simulink model "SF103A_MotRefMdl"  (R2013b)
settings: Solver=FixedStepDiscrete  StartTime=0.0  StopTime=2  FixedStep=.002  RelTol=1e-3
values from neighbouring files (symbols this model uses):
  ARCHGLBPRM_2MILLISEC_SEC_F32 = DataDict.Constant    [SF103A_MotRefMdl_DataDict.m]
  ARCHGLBPRM_2OVERSQRT3_ULS_F32 = DataDict.Constant    [SF103A_MotRefMdl_DataDict.m]
  ARCHGLBPRM_2PI_ULS_F32 = DataDict.Constant    [SF103A_MotRefMdl_DataDict.m]
  ARCHGLBPRM_4OVERSQRT3_ULS_F32 = DataDict.Constant    [SF103A_MotRefMdl_DataDict.m]
  ARCHGLBPRM_5PIOVER4_ULS_F32 = DataDict.Constant    [SF103A_MotRefMdl_DataDict.m]
  ARCHGLBPRM_FLOATZEROTHD_ULS_F32 = DataDict.Constant    [SF103A_MotRefMdl_DataDict.m]
  ARCHGLBPRM_HALFSQRT3_ULS_F32 = DataDict.Constant    [SF103A_MotRefMdl_DataDict.m]
  ARCHGLBPRM_PI_ULS_F32 = DataDict.Constant    [SF103A_MotRefMdl_DataDict.m]
  MotRefMdlCurrDaxBoostGain = DataDict.Calibration    [SF103A_MotRefMdl_DataDict.m]
  MotRefMdlCurrDaxQaxRefDelta = DataDict.Calibration    [SF103A_MotRefMdl_DataDict.m]
  MotRefMdlCurrItrnTolr = DataDict.Calibration    [SF103A_MotRefMdl_DataDict.m]
  MotRefMdlFbCtrlDi = DataDict.Calibration    [SF103A_MotRefMdl_DataDict.m]
  MotRefMdlIvtrDeadTiBrdgVltgSca = DataDict.Calibration    [SF103A_MotRefMdl_DataDict.m]
  MotRefMdlMinCurrItrnLim = DataDict.Calibration    [SF103A_MotRefMdl_DataDict.m]
  MotRefMdlMotCurrDaxMaxSca = DataDict.Calibration    [SF103A_MotRefMdl_DataDict.m]
  MotRefMdlMotVltgDerivtvTiCon = DataDict.Calibration    [SF103A_MotRefMdl_DataDict.m]
  MotRefMdlRefLocnItrnLim = DataDict.Calibration    [SF103A_MotRefMdl_DataDict.m]
  MotRefMdlTqItrnLim = DataDict.Calibration    [SF103A_MotRefMdl_DataDict.m]
  MotRefMdlTqItrnTolr = DataDict.Calibration    [SF103A_MotRefMdl_DataDict.m]
  MotRefMdlVltgModDynCmpEna = DataDict.Calibration    [SF103A_MotRefMdl_DataDict.m]
  MotRefMdlVltgOverRThdSca = DataDict.Calibration    [SF103A_MotRefMdl_DataDict.m]
  SysGlbPrmMotPoleCnt = DataDict.ImprtdCal    [SF103A_MotRefMdl_DataDict.m]
undefined symbols (not defined in the file or in its folder): MotQuad1
libraries: NxtrLim x19, simulink x4, LnrIntrpn x3, Fil x2, NxtrAbslt x2, FixdToFloat x2, FloatToFixd x2, NxtrMath x1
(part 4 of 7)

== system SF103A_MotRefMdl/MotRefMdl/MotRefMdlPer1/DAxisCurrentBoost/If Action Subsystem ==
  note: "VoltageMargin"
  note: "Vmag_min/R"
  CurrDaxMin : Inport  RequirementInfo={} %GIDa_a9cc6c0e_d971_41b8_a873_ef9f53fa8bc6
  CurrQaxMin : Inport  RequirementInfo={} %GIDa_a98a38c5_8ae3_4bcc_9086_28c16690a326  Port=2
  InterCalcns : Inport  RequirementInfo={} %GIDa_5e92023f_1a23_4fc8_ae94_2c4b8c4c5d26  Port=3
  MotTqCmdLimd : Inport  Port=4
  CurrDaxAtPeakTq : Inport  Port=5
  Action Port : ActionPort  ActionType=then
  Add : Sum  RequirementInfo={'linktype_rmi_doors' '0000bb42 (/E-STEER Core/SubSystem Specifications/Application Functions/SF99/SF103A Motor Reference Model)' '#SF103A_142' 'true' 'REQ:SF103A_142' '' } %GIDa_a7207258_8a7c_4a3a_8c14_f88ec2ccdf28
  Boost_Merge : Merge  RequirementInfo={'linktype_rmi_doors' '0000bb42 (/E-STEER Core/SubSystem Specifications/Application Functions/SF99/SF103A Motor Reference Model)' '#SF103A_145' 'true' 'REQ:SF103A_145' '' } %GIDa_8158cc00_aa92_4509_984e_a32d4237c8b1
  Bus Selector : BusSelector  RequirementInfo={} %GIDa_f3165034_7368_454c_b0f7_31404390f148  OutputSignals=VltgOverR_Ampr
  Constant : Constant  RequirementInfo={'linktype_rmi_doors' '0000bb42 (/E-STEER Core/SubSystem Specifications/Application Functions/SF99/SF103A Motor Reference Model)' '#SF103A_143' 'true' 'REQ:SF103A_143' '' } %GIDa_b9afd42a_ca58_4d6b_8dd6_d9cdb6968168  Value=MotRefMdlVltgOverRThdSca
  Constant1 : Constant  RequirementInfo={'linktype_rmi_doors' '0000bb42 (/E-STEER Core/SubSystem Specifications/Application Functions/SF99/SF103A Motor Reference Model)' '#SF103A_145' 'true' 'REQ:SF103A_145' '' } %GIDa_acfabe03_75a7_44a2_9eb9_3f49c5171f7f  Value=0  OutDataTypeStr=single
  CopyRight2 : Subsystem  Description=|  mask(Copyright Information){none=on}
      | Copyright info block.                                               
      |                                                                     
      | Place copyright information at the top of every subsystem in design.
      mask prompts: none "No parameters"
      mask help: Place copyright information at the top of every subsystem in design.
      mask Display:
      | NxtrConf = 'Nexteer Confidential';
      | 
      | sys = bdroot; %handle for the current model ("system")
      | first = get_param(sys,'Created');
      | first = first(end-3:end);  %year is last four digits
      | 
      | last = get_param(sys,'LastModifiedDate');
      | if isempty(last)
      |     last = datestr(now,'yyyy');
      | else
      |     last = last(end-3:end);
      | end
      | 
      | if strcmp(first,last)
      |     fprintf('%s -- Copyright %s Nexteer',NxtrConf,first)
      | else
      |     fprintf('%s -- %s%s- %s Nexteer',NxtrConf,char(169),first,last)
      | end
  "CurrToVoltTest " : Subsystem
  Dax_Merge : Merge  RequirementInfo={'linktype_rmi_doors' '0000bb42 (/E-STEER Core/SubSystem Specifications/Application Functions/SF99/SF103A Motor Reference Model)' '#SF103A_145' 'true' 'REQ:SF103A_145' '' } %GIDa_3f0604bd_3f78_4abe_886a_80594115c85c
  If : If  RequirementInfo={'linktype_rmi_doors' '0000bb42 (/E-STEER Core/SubSystem Specifications/Application Functions/SF99/SF103A Motor Reference Model)' '#SF103A_145' 'true' 'REQ:SF103A_145' '' ; 'linktype_rmi_doors' '0000bb42 (/E-STEER Core/SubSystem Specifications/Application Functions/SF99/SF103A Motor Reference Model)' '#SF103A_149' 'true' 'REQ:SF103A_149' '' } %GIDa_18434ab9_b410_43c2_a56e_97fbbcb99bff  IfExpression=u1 >= 0
  If Action Subsystem : Subsystem  RequirementInfo={'linktype_rmi_doors' '0000bb42 (/E-STEER Core/SubSystem Specifications/Application Functions/SF99/SF103A Motor Reference Model)' '#SF103A_149' 'true' 'REQ:SF103A_149' '' } %GIDa_5e584c9f_7420_4cd1_86a2_c32478ec1f58  TreatAsAtomicUnit=on
  Math Function : Math  RequirementInfo={'linktype_rmi_doors' '0000bb42 (/E-STEER Core/SubSystem Specifications/Application Functions/SF99/SF103A Motor Reference Model)' '#SF103A_142' 'true' 'REQ:SF103A_142' '' } %GIDa_7944bbab_6b21_43ee_b623_3ef25e5888e6  Operator=square  SaturateOnIntegerOverflow=on
  Math Function1 : Math  RequirementInfo={'linktype_rmi_doors' '0000bb42 (/E-STEER Core/SubSystem Specifications/Application Functions/SF99/SF103A Motor Reference Model)' '#SF103A_142' 'true' 'REQ:SF103A_142' '' } %GIDa_493eb05e_2677_4cd4_acc7_ad4c5e79bd89  Operator=square  SaturateOnIntegerOverflow=on
  Product : Product  RequirementInfo={'linktype_rmi_doors' '0000bb42 (/E-STEER Core/SubSystem Specifications/Application Functions/SF99/SF103A Motor Reference Model)' '#SF103A_143' 'true' 'REQ:SF103A_143' '' } %GIDa_05a785fc_6d2b_42f5_8278_a505a2fee388  RndMeth=Zero
  Qax_Merge : Merge  RequirementInfo={'linktype_rmi_doors' '0000bb42 (/E-STEER Core/SubSystem Specifications/Application Functions/SF99/SF103A Motor Reference Model)' '#SF103A_145' 'true' 'REQ:SF103A_145' '' } %GIDa_c18f4407_faf9_46c8_81f8_a25da43b62c9
  Sqrt_f32 : NxtrMath/Sqrt_f32  SFunctionSpec=single y1 = Sqrt_f32(single u1)  ShowSpec=off
      settings: AttributesFormatString=%<MaskType>
  Subtract : Sum  RequirementInfo={'linktype_rmi_doors' '0000bb42 (/E-STEER Core/SubSystem Specifications/Application Functions/SF99/SF103A Motor Reference Model)' '#SF103A_143' 'true' 'REQ:SF103A_143' '' } %GIDa_ee97ca05_4079_4b26_a98f_acc77e80c0bc  Inputs=+-
  pass_thru : Subsystem  RequirementInfo={'linktype_rmi_doors' '0000bb42 (/E-STEER Core/SubSystem Specifications/Application Functions/SF99/SF103A Motor Reference Model)' '#SF103A_145' 'true' 'REQ:SF103A_145' '' } %GIDa_4f4a4179_c5b2_4767_8ef4_f1533bcda9c5  TreatAsAtomicUnit=on
  CurrDaxBoostd : Outport  RequirementInfo={} %GIDa_c7761a80_f9a5_4df9_8815_ca0dff25a232
  CurrQaxBoostd : Outport  RequirementInfo={} %GIDa_0eb399b5_a76d_490b_968a_f2f0f65fb18a  Port=2
  BoostAmnt : Outport  RequirementInfo={} %GIDa_326380c9_363e_48c7_b65c_8aa2d98ec125  Port=3
  wires:
  Math Function1/1 -> Add/2
  Math Function/1 -> Add/1
  Sqrt_f32/1 -> Subtract/1
  Product/1 -> Subtract/2
  Add/1 -> Sqrt_f32/1  "VRBoostTotal_AmpSq"
  "CurrToVoltTest "/1(VdR_Amp) -> Math Function/1
  Subtract/1 -> If Action Subsystem/1(VRDelta), If/1  "VRDelta_Amp"
  Constant/1 -> Product/2
  "CurrToVoltTest "/2(VqR_Amp) -> Math Function1/1
  Bus Selector/1 -> Product/1  "<VltgOverR_Ampr>"
  [IqMin] -> "CurrToVoltTest "/2(IqRef_Amp)
  InterCalcns/1 -> If Action Subsystem/2(InterCalcns), Bus Selector/1, "CurrToVoltTest "/3(InterCalcns)
  MotTqCmdLimd/1 -> If Action Subsystem/4(MotTqCmdLimd)
  If/1 -> If Action Subsystem/Action
  CurrDaxAtPeakTq/1 -> If Action Subsystem/5(CurrDaxAtPeakTq)
  If/2 -> pass_thru/Action
  [IdMin] -> "CurrToVoltTest "/1(IdRef_Amp)
  CurrDaxMin/1 -> [IdMin]
  [IdMin] -> If Action Subsystem/3(CurrDaxMin)
  Constant1/1 -> pass_thru/1(In1)
  [IdMin] -> pass_thru/2(In2)
  pass_thru/1(Out1) -> Boost_Merge/1
  If Action Subsystem/1(CurrDaxBoostAmnt) -> Boost_Merge/2
  pass_thru/2(Out2) -> Dax_Merge/1
  If Action Subsystem/2(CurrDaxBoostd) -> Dax_Merge/2
  pass_thru/3(Out3) -> Qax_Merge/1
  If Action Subsystem/3(CurrQaxMin) -> Qax_Merge/2
  Dax_Merge/1 -> CurrDaxBoostd/1
  Qax_Merge/1 -> CurrQaxBoostd/1
  Boost_Merge/1 -> BoostAmnt/1
  CurrQaxMin/1 -> [IqMin]
  [IqMin] -> pass_thru/3(In3)

== system SF103A_MotRefMdl/MotRefMdl/MotRefMdlPer1/DAxisCurrentBoost/pass_thru ==
  In1 : Inport
  In2 : Inport  Port=2
  In3 : Inport  Port=3
  Action Port : ActionPort  ActionType=else
  Out1 : Outport
  Out2 : Outport  Port=2
  Out3 : Outport  Port=3
  wires:
  In1/1 -> Out1/1
  In2/1 -> Out2/1
  In3/1 -> Out3/1

== system SF103A_MotRefMdl/MotRefMdl/MotRefMdlPer1/FeedforwardVoltage/CopyRight2 ==

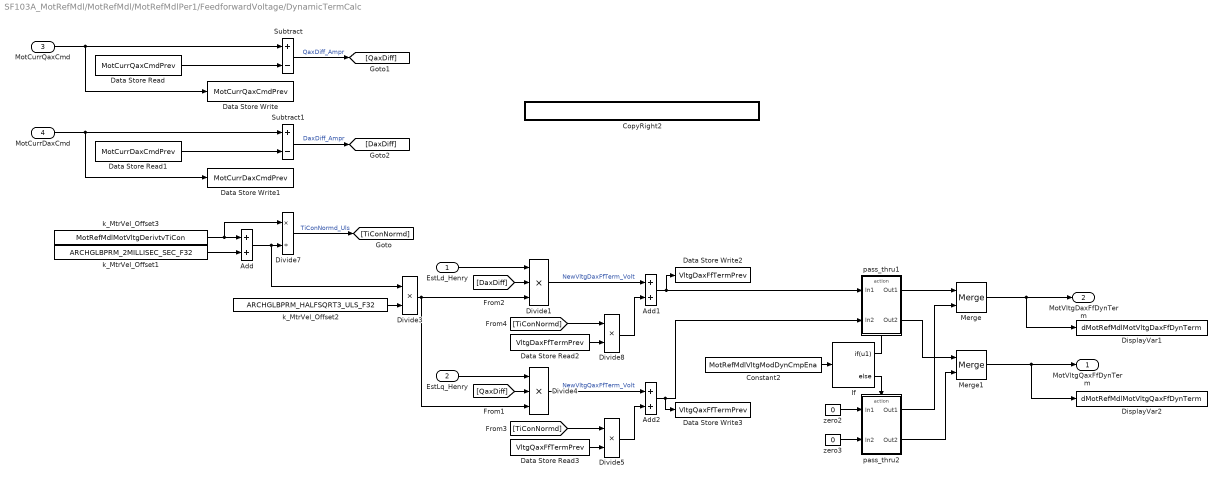
== system SF103A_MotRefMdl/MotRefMdl/MotRefMdlPer1/FeedforwardVoltage/DynamicTermCalc ==
  EstLd_Henry : Inport  RequirementInfo={} %GIDa_669719cb_8e2d_4183_8cde_e2bfb5c3b721
  EstLq_Henry : Inport  RequirementInfo={} %GIDa_1e6f10ed_a02a_410d_b0f0_b2b8d69bc7d9  Port=2
  MotCurrQaxCmd : Inport  RequirementInfo={} %GIDa_48fec4ba_508b_4013_ad2a_d4908a6c34f1  Port=3
  MotCurrDaxCmd : Inport  RequirementInfo={} %GIDa_f1550487_6b07_4eb4_b5b5_ba3d330502de  Port=4
  Add : Sum  RequirementInfo={'linktype_rmi_doors' '0000bb42 (/E-STEER Core/SubSystem Specifications/Application Functions/SF99/SF103A Motor Reference Model)' '#SF103A_160' 'true' 'REQ:SF103A_160' '' ; 'linktype_rmi_doors' '0000bb42 (/E-STEER Core/SubSystem Specifications/Application Functions/SF99/SF103A Motor Reference Model)' '#SF103A_182' 'true' 'REQ:SF103A_182' '' } %GIDa_10232317_d51a_444c_8610_964f10878767
  Add1 : Sum  RequirementInfo={'linktype_rmi_doors' '0000bb42 (/E-STEER Core/SubSystem Specifications/Application Functions/SF99/SF103A Motor Reference Model)' '#SF103A_160' 'true' 'REQ:SF103A_160' '' ; 'linktype_rmi_doors' '0000bb42 (/E-STEER Core/SubSystem Specifications/Application Functions/SF99/SF103A Motor Reference Model)' '#SF103A_182' 'true' 'REQ:SF103A_182' '' } %GIDa_669d8608_a4e4_4a27_aa85_1b2fde54e24b
  Add2 : Sum  RequirementInfo={'linktype_rmi_doors' '0000bb42 (/E-STEER Core/SubSystem Specifications/Application Functions/SF99/SF103A Motor Reference Model)' '#SF103A_160' 'true' 'REQ:SF103A_160' '' ; 'linktype_rmi_doors' '0000bb42 (/E-STEER Core/SubSystem Specifications/Application Functions/SF99/SF103A Motor Reference Model)' '#SF103A_182' 'true' 'REQ:SF103A_182' '' } %GIDa_7f87b368_be3e_4799_a4ca_a1b629f831da
  Constant2 : Constant  RequirementInfo={'linktype_rmi_doors' '0000bb42 (/E-STEER Core/SubSystem Specifications/Application Functions/SF99/SF103A Motor Reference Model)' '#SF103A_181' 'true' 'REQ:SF103A_181' '' } %GIDa_cceb1647_a34e_4756_8fd2_7c70dafabde3  Value=MotRefMdlVltgModDynCmpEna
  CopyRight2 : Subsystem  Description=|  mask(Copyright Information){none=on}
      | Copyright info block.                                               
      |                                                                     
      | Place copyright information at the top of every subsystem in design.
      mask prompts: none "No parameters"
      mask help: Place copyright information at the top of every subsystem in design.
      mask Display:
      | NxtrConf = 'Nexteer Confidential';
      | 
      | sys = bdroot; %handle for the current model ("system")
      | first = get_param(sys,'Created');
      | first = first(end-3:end);  %year is last four digits
      | 
      | last = get_param(sys,'LastModifiedDate');
      | if isempty(last)
      |     last = datestr(now,'yyyy');
      | else
      |     last = last(end-3:end);
      | end
      | 
      | if strcmp(first,last)
      |     fprintf('%s -- Copyright %s Nexteer',NxtrConf,first)
      | else
      |     fprintf('%s -- %s%s- %s Nexteer',NxtrConf,char(169),first,last)
      | end
  Data Store Read : DataStoreRead  RequirementInfo={'linktype_rmi_doors' '0000bb42 (/E-STEER Core/SubSystem Specifications/Application Functions/SF99/SF103A Motor Reference Model)' '#SF103A_160' 'true' 'REQ:SF103A_160' '' ; 'linktype_rmi_doors' '0000bb42 (/E-STEER Core/SubSystem Specifications/Application Functions/SF99/SF103A Motor Reference Model)' '#SF103A_182' 'true' 'REQ:SF103A_182' '' } %GIDa_05b9380c_f7d0_4b8b_91d2_bb3b6a9c7c49  Priority=1  DataStoreName=MotCurrQaxCmdPrev
      settings: AttributesFormatString="priority:  %<Priority>"
  Data Store Read1 : DataStoreRead  RequirementInfo={'linktype_rmi_doors' '0000bb42 (/E-STEER Core/SubSystem Specifications/Application Functions/SF99/SF103A Motor Reference Model)' '#SF103A_160' 'true' 'REQ:SF103A_160' '' ; 'linktype_rmi_doors' '0000bb42 (/E-STEER Core/SubSystem Specifications/Application Functions/SF99/SF103A Motor Reference Model)' '#SF103A_182' 'true' 'REQ:SF103A_182' '' } %GIDa_c3acf00d_65c5_46ce_8b95_f1a4693b3fea  Priority=1  DataStoreName=MotCurrDaxCmdPrev
      settings: AttributesFormatString="priority:  %<Priority>"
  Data Store Read2 : DataStoreRead  RequirementInfo={'linktype_rmi_doors' '0000bb42 (/E-STEER Core/SubSystem Specifications/Application Functions/SF99/SF103A Motor Reference Model)' '#SF103A_160' 'true' 'REQ:SF103A_160' '' ; 'linktype_rmi_doors' '0000bb42 (/E-STEER Core/SubSystem Specifications/Application Functions/SF99/SF103A Motor Reference Model)' '#SF103A_182' 'true' 'REQ:SF103A_182' '' } %GIDa_cb6238cf_a10b_4525_b339_784cfc00b0f8  DataStoreName=VltgDaxFfTermPrev
  Data Store Read3 : DataStoreRead  RequirementInfo={'linktype_rmi_doors' '0000bb42 (/E-STEER Core/SubSystem Specifications/Application Functions/SF99/SF103A Motor Reference Model)' '#SF103A_160' 'true' 'REQ:SF103A_160' '' ; 'linktype_rmi_doors' '0000bb42 (/E-STEER Core/SubSystem Specifications/Application Functions/SF99/SF103A Motor Reference Model)' '#SF103A_182' 'true' 'REQ:SF103A_182' '' } %GIDa_371f5c13_60a5_488d_aaed_0ad251289211  DataStoreName=VltgQaxFfTermPrev
  Data Store Write : DataStoreWrite  RequirementInfo={'linktype_rmi_doors' '0000bb42 (/E-STEER Core/SubSystem Specifications/Application Functions/SF99/SF103A Motor Reference Model)' '#SF103A_160' 'true' 'REQ:SF103A_160' '' ; 'linktype_rmi_doors' '0000bb42 (/E-STEER Core/SubSystem Specifications/Application Functions/SF99/SF103A Motor Reference Model)' '#SF103A_182' 'true' 'REQ:SF103A_182' '' } %GIDa_46d73cb8_92af_44e2_bd02_5d5bfdf03e86  Priority=2  DataStoreName=MotCurrQaxCmdPrev
      settings: AttributesFormatString="priority:  %<Priority>"
  Data Store Write1 : DataStoreWrite  RequirementInfo={'linktype_rmi_doors' '0000bb42 (/E-STEER Core/SubSystem Specifications/Application Functions/SF99/SF103A Motor Reference Model)' '#SF103A_160' 'true' 'REQ:SF103A_160' '' ; 'linktype_rmi_doors' '0000bb42 (/E-STEER Core/SubSystem Specifications/Application Functions/SF99/SF103A Motor Reference Model)' '#SF103A_182' 'true' 'REQ:SF103A_182' '' } %GIDa_222fdf85_f65f_4ac2_be52_2e256b249118  Priority=2  DataStoreName=MotCurrDaxCmdPrev
      settings: AttributesFormatString="priority:  %<Priority>"
  Data Store Write2 : DataStoreWrite  RequirementInfo={'linktype_rmi_doors' '0000bb42 (/E-STEER Core/SubSystem Specifications/Application Functions/SF99/SF103A Motor Reference Model)' '#SF103A_160' 'true' 'REQ:SF103A_160' '' ; 'linktype_rmi_doors' '0000bb42 (/E-STEER Core/SubSystem Specifications/Application Functions/SF99/SF103A Motor Reference Model)' '#SF103A_182' 'true' 'REQ:SF103A_182' '' } %GIDa_e2c90ff9_8f16_41a4_9d01_099185af077c  DataStoreName=VltgDaxFfTermPrev
  Data Store Write3 : DataStoreWrite  RequirementInfo={'linktype_rmi_doors' '0000bb42 (/E-STEER Core/SubSystem Specifications/Application Functions/SF99/SF103A Motor Reference Model)' '#SF103A_160' 'true' 'REQ:SF103A_160' '' ; 'linktype_rmi_doors' '0000bb42 (/E-STEER Core/SubSystem Specifications/Application Functions/SF99/SF103A Motor Reference Model)' '#SF103A_182' 'true' 'REQ:SF103A_182' '' } %GIDa_0162ae4b_0c49_489b_aeca_a87d5659adf4  DataStoreName=VltgQaxFfTermPrev
  DisplayVar1 : DataStoreWrite  DataStoreName=dMotRefMdlMotVltgDaxFfDynTerm
  DisplayVar2 : DataStoreWrite  DataStoreName=dMotRefMdlMotVltgQaxFfDynTerm
  Divide1 : Product  RequirementInfo={'linktype_rmi_doors' '0000bb42 (/E-STEER Core/SubSystem Specifications/Application Functions/SF99/SF103A Motor Reference Model)' '#SF103A_160' 'true' 'REQ:SF103A_160' '' ; 'linktype_rmi_doors' '0000bb42 (/E-STEER Core/SubSystem Specifications/Application Functions/SF99/SF103A Motor Reference Model)' '#SF103A_182' 'true' 'REQ:SF103A_182' '' } %GIDa_e0d481e1_9aed_48d8_b95d_d63f79d4ba76  Inputs=3
  Divide3 : Product  RequirementInfo={'linktype_rmi_doors' '0000bb42 (/E-STEER Core/SubSystem Specifications/Application Functions/SF99/SF103A Motor Reference Model)' '#SF103A_160' 'true' 'REQ:SF103A_160' '' ; 'linktype_rmi_doors' '0000bb42 (/E-STEER Core/SubSystem Specifications/Application Functions/SF99/SF103A Motor Reference Model)' '#SF103A_182' 'true' 'REQ:SF103A_182' '' } %GIDa_7eb71138_5e12_421b_b02e_711bd10f8c27
  Divide4 : Product  RequirementInfo={'linktype_rmi_doors' '0000bb42 (/E-STEER Core/SubSystem Specifications/Application Functions/SF99/SF103A Motor Reference Model)' '#SF103A_160' 'true' 'REQ:SF103A_160' '' ; 'linktype_rmi_doors' '0000bb42 (/E-STEER Core/SubSystem Specifications/Application Functions/SF99/SF103A Motor Reference Model)' '#SF103A_182' 'true' 'REQ:SF103A_182' '' } %GIDa_f993f8e8_eee0_4f2a_98e0_d3406be52488  Inputs=3
  Divide5 : Product  RequirementInfo={'linktype_rmi_doors' '0000bb42 (/E-STEER Core/SubSystem Specifications/Application Functions/SF99/SF103A Motor Reference Model)' '#SF103A_160' 'true' 'REQ:SF103A_160' '' ; 'linktype_rmi_doors' '0000bb42 (/E-STEER Core/SubSystem Specifications/Application Functions/SF99/SF103A Motor Reference Model)' '#SF103A_182' 'true' 'REQ:SF103A_182' '' } %GIDa_68c6400c_dcf8_47b2_8553_e7e58ff640ab
  Divide7 : Product  RequirementInfo={'linktype_rmi_doors' '0000bb42 (/E-STEER Core/SubSystem Specifications/Application Functions/SF99/SF103A Motor Reference Model)' '#SF103A_160' 'true' 'REQ:SF103A_160' '' ; 'linktype_rmi_doors' '0000bb42 (/E-STEER Core/SubSystem Specifications/Application Functions/SF99/SF103A Motor Reference Model)' '#SF103A_182' 'true' 'REQ:SF103A_182' '' } %GIDa_9a02108e_1cb2_44ec_89b4_df7ca7f60ec4  Inputs=*/
  Divide8 : Product  RequirementInfo={'linktype_rmi_doors' '0000bb42 (/E-STEER Core/SubSystem Specifications/Application Functions/SF99/SF103A Motor Reference Model)' '#SF103A_160' 'true' 'REQ:SF103A_160' '' ; 'linktype_rmi_doors' '0000bb42 (/E-STEER Core/SubSystem Specifications/Application Functions/SF99/SF103A Motor Reference Model)' '#SF103A_182' 'true' 'REQ:SF103A_182' '' } %GIDa_f2450640_a176_4b67_8e11_053e0b7e319f
  If : If  RequirementInfo={'linktype_rmi_doors' '0000bb42 (/E-STEER Core/SubSystem Specifications/Application Functions/SF99/SF103A Motor Reference Model)' '#SF103A_181' 'true' 'REQ:SF103A_181' '' } %GIDa_744f793a_5a96_49e2_9cd0_9a2c1bea1fce  IfExpression=u1
  Merge : Merge  RequirementInfo={'linktype_rmi_doors' '0000bb42 (/E-STEER Core/SubSystem Specifications/Application Functions/SF99/SF103A Motor Reference Model)' '#SF103A_181' 'true' 'REQ:SF103A_181' '' } %GIDa_04ad99a4_ff32_4b1c_b335_6a7ec2ed5ec1
  Merge1 : Merge  RequirementInfo={'linktype_rmi_doors' '0000bb42 (/E-STEER Core/SubSystem Specifications/Application Functions/SF99/SF103A Motor Reference Model)' '#SF103A_181' 'true' 'REQ:SF103A_181' '' } %GIDa_1a839eab_9789_44ee_9126_b9e8e970b4c4
  Subtract : Sum  RequirementInfo={'linktype_rmi_doors' '0000bb42 (/E-STEER Core/SubSystem Specifications/Application Functions/SF99/SF103A Motor Reference Model)' '#SF103A_160' 'true' 'REQ:SF103A_160' '' ; 'linktype_rmi_doors' '0000bb42 (/E-STEER Core/SubSystem Specifications/Application Functions/SF99/SF103A Motor Reference Model)' '#SF103A_182' 'true' 'REQ:SF103A_182' '' } %GIDa_1270906d_c7ff_45d2_960f_0000ee2a3a50  Inputs=+-
  Subtract1 : Sum  RequirementInfo={'linktype_rmi_doors' '0000bb42 (/E-STEER Core/SubSystem Specifications/Application Functions/SF99/SF103A Motor Reference Model)' '#SF103A_160' 'true' 'REQ:SF103A_160' '' ; 'linktype_rmi_doors' '0000bb42 (/E-STEER Core/SubSystem Specifications/Application Functions/SF99/SF103A Motor Reference Model)' '#SF103A_182' 'true' 'REQ:SF103A_182' '' } %GIDa_963030ea_bc3e_4fe2_8de1_76f630906100  Inputs=+-
  k_MtrVel_Offset1 : Constant  RequirementInfo={'linktype_rmi_doors' '0000bb42 (/E-STEER Core/SubSystem Specifications/Application Functions/SF99/SF103A Motor Reference Model)' '#SF103A_160' 'true' 'REQ:SF103A_160' '' ; 'linktype_rmi_doors' '0000bb42 (/E-STEER Core/SubSystem Specifications/Application Functions/SF99/SF103A Motor Reference Model)' '#SF103A_182' 'true' 'REQ:SF103A_182' '' } %GIDa_1e8eefaf_7d7a_43ec_a530_2638852dc221  Value=ARCHGLBPRM_2MILLISEC_SEC_F32  SampleTime=-1
  k_MtrVel_Offset2 : Constant  RequirementInfo={'linktype_rmi_doors' '0000bb42 (/E-STEER Core/SubSystem Specifications/Application Functions/SF99/SF103A Motor Reference Model)' '#SF103A_160' 'true' 'REQ:SF103A_160' '' ; 'linktype_rmi_doors' '0000bb42 (/E-STEER Core/SubSystem Specifications/Application Functions/SF99/SF103A Motor Reference Model)' '#SF103A_182' 'true' 'REQ:SF103A_182' '' } %GIDa_9417c886_04ae_4f0a_963d_bb2689337753  Value=ARCHGLBPRM_HALFSQRT3_ULS_F32  SampleTime=-1
  k_MtrVel_Offset3 : Constant  RequirementInfo={'linktype_rmi_doors' '0000bb42 (/E-STEER Core/SubSystem Specifications/Application Functions/SF99/SF103A Motor Reference Model)' '#SF103A_160' 'true' 'REQ:SF103A_160' '' ; 'linktype_rmi_doors' '0000bb42 (/E-STEER Core/SubSystem Specifications/Application Functions/SF99/SF103A Motor Reference Model)' '#SF103A_182' 'true' 'REQ:SF103A_182' '' } %GIDa_b9dc4d85_a64a_4da0_9f5e_3e78d687d8c3  Value=MotRefMdlMotVltgDerivtvTiCon  SampleTime=-1
  pass_thru1 : Subsystem  RequirementInfo={'linktype_rmi_doors' '0000bb42 (/E-STEER Core/SubSystem Specifications/Application Functions/SF99/SF103A Motor Reference Model)' '#SF103A_181' 'true' 'REQ:SF103A_181' '' } %GIDa_d39f690c_ffc6_4c9a_a69f_e3441288fc74  TreatAsAtomicUnit=on
  pass_thru2 : Subsystem  RequirementInfo={'linktype_rmi_doors' '0000bb42 (/E-STEER Core/SubSystem Specifications/Application Functions/SF99/SF103A Motor Reference Model)' '#SF103A_181' 'true' 'REQ:SF103A_181' '' } %GIDa_9db7dfbc_fc11_499c_bcac_72f4528c9821  TreatAsAtomicUnit=on
  zero2 : Constant  RequirementInfo={'linktype_rmi_doors' '0000bb42 (/E-STEER Core/SubSystem Specifications/Application Functions/SF99/SF103A Motor Reference Model)' '#SF103A_181' 'true' 'REQ:SF103A_181' '' } %GIDa_dee8525e_7980_4645_a100_3343d99c3ea6  Value=0  OutDataTypeStr=single
  zero3 : Constant  RequirementInfo={'linktype_rmi_doors' '0000bb42 (/E-STEER Core/SubSystem Specifications/Application Functions/SF99/SF103A Motor Reference Model)' '#SF103A_181' 'true' 'REQ:SF103A_181' '' } %GIDa_5afe63be_75e4_4e82_a301_20ee1799dd09  Value=0  OutDataTypeStr=single
  MotVltgQaxFfDynTerm : Outport  RequirementInfo={} %GIDa_4923439f_da37_4deb_b8f0_ad8b4f8cb4a2
  MotVltgDaxFfDynTerm : Outport  RequirementInfo={} %GIDa_2eb69af5_3e2b_415c_aa7c_6a063f99d234  Port=2
  wires:
  Add2/1 -> pass_thru1/2(In2), Data Store Write3/1
  k_MtrVel_Offset2/1 -> Divide3/2
  Divide4/1 -> Add2/1  "NewVltgQaxFfTerm_Volt"
  MotCurrQaxCmd/1 -> Subtract/1, Data Store Write/1
  Data Store Read/1 -> Subtract/2
  MotCurrDaxCmd/1 -> Data Store Write1/1, Subtract1/1
  [DaxDiff] -> Divide1/2
  Divide5/1 -> Add2/2
  Data Store Read3/1 -> Divide5/2
  Divide1/1 -> Add1/1  "NewVltgDaxFfTerm_Volt"
  Data Store Read2/1 -> Divide8/2
  Divide8/1 -> Add1/2
  Add1/1 -> Data Store Write2/1, pass_thru1/1(In1)
  Merge1/1 -> DisplayVar2/1, MotVltgQaxFfDynTerm/1
  Merge/1 -> DisplayVar1/1, MotVltgDaxFfDynTerm/1
  Data Store Read1/1 -> Subtract1/2
  Divide7/1 -> [TiConNormd]  "TiConNormd_Uls"
  Divide3/1 -> Divide4/3, Divide1/3
  [TiConNormd] -> Divide5/1
  [TiConNormd] -> Divide8/1
  k_MtrVel_Offset3/1 -> Divide7/1, Add/1
  k_MtrVel_Offset1/1 -> Add/2
  Add/1 -> Divide3/1, Divide7/2
  Subtract/1 -> [QaxDiff]  "QaxDiff_Ampr"
  EstLq_Henry/1 -> Divide4/1
  [QaxDiff] -> Divide4/2
  Subtract1/1 -> [DaxDiff]  "DaxDiff_Ampr"
  EstLd_Henry/1 -> Divide1/1
  If/1 -> pass_thru1/Action
  If/2 -> pass_thru2/Action
  Constant2/1 -> If/1
  zero3/1 -> pass_thru2/2(In2)
  zero2/1 -> pass_thru2/1(In1)
  pass_thru1/1(Out1) -> Merge/1
  pass_thru2/1(Out1) -> Merge/2
  pass_thru1/2(Out2) -> Merge1/1
  pass_thru2/2(Out2) -> Merge1/2

== system SF103A_MotRefMdl/MotRefMdl/MotRefMdlPer1/FeedforwardVoltage/FeedforwardSelection ==
  MotVltgDaxFfStat : Inport  RequirementInfo={} %GIDa_4ed36d18_6fc6_454d_91a6_26085fefa5da
  MotVltgQaxFfStat : Inport  RequirementInfo={} %GIDa_fa3af2bc_548c_4a58_9d9d_6fb3b743484b  Port=2
  CurrMeasLoaMtgtnEna : Inport  RequirementInfo={} %GIDa_8f665609_c073_4ded_8f96_8b49bf08bbcd  Port=3
  IvtrLoaMtgtnEn : Inport  RequirementInfo={} %GIDa_ee78e044_3616_4a16_8e7d_09b6d0e76cc8  Port=4
  MotVltgQaxFfDynTerm : Inport  RequirementInfo={} %GIDa_ecdd0ce4_fd73_44d0_bb5b_e9a916e4481b  Port=5
  MotVltgDaxFfDynTerm : Inport  RequirementInfo={} %GIDa_20ae9a13_367e_461b_8361_ebdfedc23ab6  Port=6
  InterCalcns : Inport  RequirementInfo={} %GIDa_17cb2d5b_fa5c_45da_be0c_54c6362108d4  Port=7
  DualEcuMotCtrlMtgtnEna : Inport  RequirementInfo={'linktype_rmi_doors' '0000bb42 (/E-STEER Core/SubSystem Specifications/Application Functions/SF99/SF103A Motor Reference Model)' '#SF103A_36' 'true' 'REQ:SF103A_36' '' } %GIDa_dcf1a5c0_6f7a_47d6_b99a_5704408dc385  Port=8
  Add : Sum  RequirementInfo={'linktype_rmi_doors' '0000bb42 (/E-STEER Core/SubSystem Specifications/Application Functions/SF99/SF103A Motor Reference Model)' '#SF103A_161' 'true' 'REQ:SF103A_161' '' ; 'linktype_rmi_doors' '0000bb42 (/E-STEER Core/SubSystem Specifications/Application Functions/SF99/SF103A Motor Reference Model)' '#SF103A_162' 'true' 'REQ:SF103A_162' '' } %GIDa_eedfce42_4b69_4d58_ae59_551ad81857c2
  Add1 : Sum  RequirementInfo={'linktype_rmi_doors' '0000bb42 (/E-STEER Core/SubSystem Specifications/Application Functions/SF99/SF103A Motor Reference Model)' '#SF103A_161' 'true' 'REQ:SF103A_161' '' ; 'linktype_rmi_doors' '0000bb42 (/E-STEER Core/SubSystem Specifications/Application Functions/SF99/SF103A Motor Reference Model)' '#SF103A_162' 'true' 'REQ:SF103A_162' '' } %GIDa_7b665e68_ec84_46c0_81a0_54cc5d3deb60
  CopyRight2 : Subsystem  Description=|  mask(Copyright Information){none=on}
      | Copyright info block.                                               
      |                                                                     
      | Place copyright information at the top of every subsystem in design.
      mask prompts: none "No parameters"
      mask help: Place copyright information at the top of every subsystem in design.
      mask Display:
      | NxtrConf = 'Nexteer Confidential';
      | 
      | sys = bdroot; %handle for the current model ("system")
      | first = get_param(sys,'Created');
      | first = first(end-3:end);  %year is last four digits
      | 
      | last = get_param(sys,'LastModifiedDate');
      | if isempty(last)
      |     last = datestr(now,'yyyy');
      | else
      |     last = last(end-3:end);
      | end
      | 
      | if strcmp(first,last)
      |     fprintf('%s -- Copyright %s Nexteer',NxtrConf,first)
      | else
      |     fprintf('%s -- %s%s- %s Nexteer',NxtrConf,char(169),first,last)
      | end
  DisplayVar1 : DataStoreWrite  RequirementInfo={'linktype_rmi_doors' '0000bb42 (/E-STEER Core/SubSystem Specifications/Application Functions/SF99/SF103A Motor Reference Model)' '#SF103A_162' 'true' 'REQ:SF103A_162' '' } %GIDa_75616f26_dcff_4d96_80c1_43492b9716ab  DataStoreName=dMotRefMdlMotVltgDaxFfDyn
  DisplayVar2 : DataStoreWrite  RequirementInfo={'linktype_rmi_doors' '0000bb42 (/E-STEER Core/SubSystem Specifications/Application Functions/SF99/SF103A Motor Reference Model)' '#SF103A_162' 'true' 'REQ:SF103A_162' '' } %GIDa_2d73536a_b1c3_488e_87b8_73dafe3ada2d  DataStoreName=dMotRefMdlMotVltgQaxFfDyn
  Merge : Merge  RequirementInfo={'linktype_rmi_doors' '0000bb42 (/E-STEER Core/SubSystem Specifications/Application Functions/SF99/SF103A Motor Reference Model)' '#SF103A_162' 'true' 'REQ:SF103A_162' '' } %GIDa_916cd493_c92f_43a0_a74a_208fdef1e086
  Merge1 : Merge  RequirementInfo={'linktype_rmi_doors' '0000bb42 (/E-STEER Core/SubSystem Specifications/Application Functions/SF99/SF103A Motor Reference Model)' '#SF103A_162' 'true' 'REQ:SF103A_162' '' } %GIDa_0704bc3d_e1f7_4dbb_8492_567d39169c1e
  VltgModOperSel_If : If  RequirementInfo={'linktype_rmi_doors' '0000bb42 (/E-STEER Core/SubSystem Specifications/Application Functions/SF99/SF103A Motor Reference Model)' '#SF103A_163' 'true' 'REQ:SF103A_163' '' ; 'linktype_rmi_doors' '0000bb42 (/E-STEER Core/SubSystem Specifications/Application Functions/SF99/SF103A Motor Reference Model)' '#SF103A_162' 'true' 'REQ:SF103A_162' '' } %GIDa_07e966fb_c4d5_49d6_99b8_1705a5c904fd  NumInputs=4  IfExpression=u1|u2|u3|u4
  k_MtrVel_Offset9 : Constant  RequirementInfo={'linktype_rmi_doors' '0000bb42 (/E-STEER Core/SubSystem Specifications/Application Functions/SF99/SF103A Motor Reference Model)' '#SF103A_163' 'true' 'REQ:SF103A_163' '' ; 'linktype_rmi_doors' '0000bb42 (/E-STEER Core/SubSystem Specifications/Application Functions/SF99/SF103A Motor Reference Model)' '#SF103A_162' 'true' 'REQ:SF103A_162' '' } %GIDa_2d6308fc_acb0_437b_bb55_8b4034cad9d8  Value=MotRefMdlFbCtrlDi  SampleTime=-1
  pass_thru1 : Subsystem  RequirementInfo={'linktype_rmi_doors' '0000bb42 (/E-STEER Core/SubSystem Specifications/Application Functions/SF99/SF103A Motor Reference Model)' '#SF103A_162' 'true' 'REQ:SF103A_162' '' } %GIDa_9cc8fc51_68ec_439b_a285_693108941e78  TreatAsAtomicUnit=on
  pass_thru2 : Subsystem  RequirementInfo={'linktype_rmi_doors' '0000bb42 (/E-STEER Core/SubSystem Specifications/Application Functions/SF99/SF103A Motor Reference Model)' '#SF103A_162' 'true' 'REQ:SF103A_162' '' } %GIDa_eea92d70_5a4a_4d19_a908_87a256cafd47  TreatAsAtomicUnit=on
  zero : Constant  RequirementInfo={'linktype_rmi_doors' '0000bb42 (/E-STEER Core/SubSystem Specifications/Application Functions/SF99/SF103A Motor Reference Model)' '#SF103A_162' 'true' 'REQ:SF103A_162' '' } %GIDa_19b7484b_479d_4dae_b3e8_de7d5ae084c5  Value=0  OutDataTypeStr=single  SampleTime=-1
  MotVltgDaxFf : Outport  RequirementInfo={} %GIDa_9734aed4_47c2_4464_920f_e1453441c511
  MotVltgQaxFf : Outport  RequirementInfo={} %GIDa_083190bb_5dc5_443e_a91c_cb729cebc8dc  Port=2
  wires:
  Add/1 -> DisplayVar1/1, pass_thru1/1(In1)
  Add1/1 -> DisplayVar2/1, pass_thru1/2(In2)
  MotVltgDaxFfStat/1 -> Add/1
  MotVltgDaxFfDynTerm/1 -> Add/2
  MotVltgQaxFfDynTerm/1 -> Add1/2
  MotVltgQaxFfStat/1 -> Add1/1
  CurrMeasLoaMtgtnEna/1 -> VltgModOperSel_If/1
  IvtrLoaMtgtnEn/1 -> VltgModOperSel_If/2
  k_MtrVel_Offset9/1 -> VltgModOperSel_If/3
  zero/1 -> pass_thru2/1(In1)
  VltgModOperSel_If/2 -> pass_thru2/Action
  VltgModOperSel_If/1 -> pass_thru1/Action
  Merge/1 -> MotVltgQaxFf/1
  Merge1/1 -> MotVltgDaxFf/1
  pass_thru1/1(Out1) -> Merge1/1
  pass_thru2/1(Out1) -> Merge1/2
  pass_thru1/2(Out2) -> Merge/1
  pass_thru2/2(Out2) -> Merge/2
  DualEcuMotCtrlMtgtnEna/1 -> VltgModOperSel_If/4
  InterCalcns/1 -> pass_thru2/2(In2)

== system SF103A_MotRefMdl/MotRefMdl/MotRefMdlPer1/IntermediateCalculations/CopyRight2 ==

== system SF103A_MotRefMdl/MotRefMdl/MotRefMdlPer1/LocateRef/CopyRight2 ==

== system SF103A_MotRefMdl/MotRefMdl/MotRefMdlPer1/LocateRef/F_CalcIqCmd_1 ==
  MotTqCmd : Inport  RequirementInfo={} %GIDa_0ab27989_e69c_4753_9494_79dc9cff73ee
  CurrDaxMax : Inport  RequirementInfo={} %GIDa_7afc7db3_9efb_4349_810d_1f5cb6fc8d00  Port=2
  InterCalcns : Inport  RequirementInfo={} %GIDa_42ab200f_4815_4b0f_ad20_6051d13ef1d1  Port=3
  Add : Sum  RequirementInfo={'linktype_rmi_doors' '0000bb42 (/E-STEER Core/SubSystem Specifications/Application Functions/SF99/SF103A Motor Reference Model)' '#SF103A_115' 'true' 'REQ:SF103A_115' '' } %GIDa_aab15ed7_4aee_46c0_a29b_59804a067df0
  Bus Selector : BusSelector  RequirementInfo={} %GIDa_6194c0ef_872b_450f_be5a_0672122f9642  OutputSignals=Ke_VoltPerRadPerSec,RelncTqCoeff_Henry_f32
  CopyRight2 : Subsystem  Description=|  mask(Copyright Information){none=on}
      | Copyright info block.                                               
      |                                                                     
      | Place copyright information at the top of every subsystem in design.
      mask prompts: none "No parameters"
      mask help: Place copyright information at the top of every subsystem in design.
      mask Display:
      | NxtrConf = 'Nexteer Confidential';
      | 
      | sys = bdroot; %handle for the current model ("system")
      | first = get_param(sys,'Created');
      | first = first(end-3:end);  %year is last four digits
      | 
      | last = get_param(sys,'LastModifiedDate');
      | if isempty(last)
      |     last = datestr(now,'yyyy');
      | else
      |     last = last(end-3:end);
      | end
      | 
      | if strcmp(first,last)
      |     fprintf('%s -- Copyright %s Nexteer',NxtrConf,first)
      | else
      |     fprintf('%s -- %s%s- %s Nexteer',NxtrConf,char(169),first,last)
      | end
  Product : Product  RequirementInfo={'linktype_rmi_doors' '0000bb42 (/E-STEER Core/SubSystem Specifications/Application Functions/SF99/SF103A Motor Reference Model)' '#SF103A_115' 'true' 'REQ:SF103A_115' '' } %GIDa_9649270f_c377_4e1b_9787_16ef90a01cb3  RndMeth=Zero
  Product1 : Product  RequirementInfo={'linktype_rmi_doors' '0000bb42 (/E-STEER Core/SubSystem Specifications/Application Functions/SF99/SF103A Motor Reference Model)' '#SF103A_115' 'true' 'REQ:SF103A_115' '' } %GIDa_63edbcc7_d999_4d55_b8d2_02dbcd8c4b86  Inputs=*/  RndMeth=Zero
  CurrQaxMax : Outport  RequirementInfo={} %GIDa_c7383983_8e5b_4ae2_9f78_57c8f6f22687
  wires:
  Product1/1 -> CurrQaxMax/1
  MotTqCmd/1 -> Product1/1
  Add/1 -> Product1/2
  Bus Selector/1 -> Add/1  "<Ke_VoltPerRadPerSec>"
  CurrDaxMax/1 -> Product/2
  Bus Selector/2 -> Product/1  "<RelncTqCoeff_Henry_f32>"
  InterCalcns/1 -> Bus Selector/1
  Product/1 -> Add/2

== system SF103A_MotRefMdl/MotRefMdl/MotRefMdlPer1/LocateRef/F_ItoV_1  ==
  IdRef_Amp : Inport  RequirementInfo={} %GIDa_78168ed3_74de_42ca_910c_bd14fa523647
  IqRef_Amp : Inport  RequirementInfo={} %GIDa_a7516f4f_243e_4d41_bf3f_3dd1437d8cc7  Port=2
  IntermediateCalcs : Inport  RequirementInfo={} %GIDa_fe03aba2_e681_4535_9fb6_2a7c7d629df6  Port=3
  Add : Sum  RequirementInfo={'linktype_rmi_doors' '0000bb42 (/E-STEER Core/SubSystem Specifications/Application Functions/SF99/SF103A Motor Reference Model)' '#SF103A_116' 'true' 'REQ:SF103A_116' '' } %GIDa_26f470b6_c6b6_4a34_b0f9_9a59433055d5  Inputs=+++
  Bus Selector1 : BusSelector  RequirementInfo={} %GIDa_01c83717_e8c0_4f13_abf5_13e70d355ae7  OutputSignals=ReacncQaxOverR,ReacncDaxOverR,EgOverR_Ampr
  CopyRight2 : Subsystem  Description=|  mask(Copyright Information){none=on}
      | Copyright info block.                                               
      |                                                                     
      | Place copyright information at the top of every subsystem in design.
      mask prompts: none "No parameters"
      mask help: Place copyright information at the top of every subsystem in design.
      mask Display:
      | NxtrConf = 'Nexteer Confidential';
      | 
      | sys = bdroot; %handle for the current model ("system")
      | first = get_param(sys,'Created');
      | first = first(end-3:end);  %year is last four digits
      | 
      | last = get_param(sys,'LastModifiedDate');
      | if isempty(last)
      |     last = datestr(now,'yyyy');
      | else
      |     last = last(end-3:end);
      | end
      | 
      | if strcmp(first,last)
      |     fprintf('%s -- Copyright %s Nexteer',NxtrConf,first)
      | else
      |     fprintf('%s -- %s%s- %s Nexteer',NxtrConf,char(169),first,last)
      | end
  Product : Product  RequirementInfo={'linktype_rmi_doors' '0000bb42 (/E-STEER Core/SubSystem Specifications/Application Functions/SF99/SF103A Motor Reference Model)' '#SF103A_116' 'true' 'REQ:SF103A_116' '' } %GIDa_2898b8af_0e80_4ea0_83ad_1dea7f56f62c  RndMeth=Zero
  Product1 : Product  RequirementInfo={'linktype_rmi_doors' '0000bb42 (/E-STEER Core/SubSystem Specifications/Application Functions/SF99/SF103A Motor Reference Model)' '#SF103A_116' 'true' 'REQ:SF103A_116' '' } %GIDa_627d022f_22b4_4049_88b0_64f8bc4b0bf4  RndMeth=Zero
  Subtract : Sum  RequirementInfo={'linktype_rmi_doors' '0000bb42 (/E-STEER Core/SubSystem Specifications/Application Functions/SF99/SF103A Motor Reference Model)' '#SF103A_116' 'true' 'REQ:SF103A_116' '' } %GIDa_120396b6_f836_44a1_9ee1_450cff0d1a7a  Inputs=+-
  VdR_Amp : Outport  RequirementInfo={} %GIDa_21621110_c272_4604_9470_844af3215089
  VqR_Amp : Outport  RequirementInfo={} %GIDa_160d2d1d_2485_48db_9c8d_18923ecd7d23  Port=2
  wires:
  IqRef_Amp/1 -> Add/1, Product/1
  IdRef_Amp/1 -> Subtract/2, Product1/1
  IntermediateCalcs/1 -> Bus Selector1/1
  Bus Selector1/1 -> Product/2  "<ReacncQaxOverR>"
  Bus Selector1/2 -> Product1/2  "<ReacncDaxOverR>"
  Bus Selector1/3 -> Add/3  "<EgOverR_Ampr>"
  Product/1 -> Subtract/1
  Subtract/1 -> VdR_Amp/1
  Product1/1 -> Add/2
  Add/1 -> VqR_Amp/1

== system SF103A_MotRefMdl/MotRefMdl/MotRefMdlPer1/LocateRef/F_ItoV_2 ==
  IdRef_Amp : Inport  RequirementInfo={} %GIDa_764cea99_7ded_4e24_ab1f_fab9acadece6
  IqRef_Amp : Inport  RequirementInfo={} %GIDa_da4130fa_5848_4b9c_8cdd_aae9ddeeb9e8  Port=2
  IntermediateCalcs : Inport  RequirementInfo={} %GIDa_7add00f5_d91b_439e_8285_4169ff834451  Port=3
  Add : Sum  RequirementInfo={'linktype_rmi_doors' '0000bb42 (/E-STEER Core/SubSystem Specifications/Application Functions/SF99/SF103A Motor Reference Model)' '#SF103A_116' 'true' 'REQ:SF103A_116' '' } %GIDa_2ca70198_7786_4060_81a1_221a302d27f4  Inputs=+++
  Bus Selector1 : BusSelector  RequirementInfo={} %GIDa_73f4aac6_e4b2_41f3_90e0_e7860ddd1da8  OutputSignals=ReacncQaxOverR,ReacncDaxOverR,EgOverR_Ampr
  CopyRight2 : Subsystem  Description=|  mask(Copyright Information){none=on}
      | Copyright info block.                                               
      |                                                                     
      | Place copyright information at the top of every subsystem in design.
      mask prompts: none "No parameters"
      mask help: Place copyright information at the top of every subsystem in design.
      mask Display:
      | NxtrConf = 'Nexteer Confidential';
      | 
      | sys = bdroot; %handle for the current model ("system")
      | first = get_param(sys,'Created');
      | first = first(end-3:end);  %year is last four digits
      | 
      | last = get_param(sys,'LastModifiedDate');
      | if isempty(last)
      |     last = datestr(now,'yyyy');
      | else
      |     last = last(end-3:end);
      | end
      | 
      | if strcmp(first,last)
      |     fprintf('%s -- Copyright %s Nexteer',NxtrConf,first)
      | else
      |     fprintf('%s -- %s%s- %s Nexteer',NxtrConf,char(169),first,last)
      | end
  Product : Product  RequirementInfo={'linktype_rmi_doors' '0000bb42 (/E-STEER Core/SubSystem Specifications/Application Functions/SF99/SF103A Motor Reference Model)' '#SF103A_116' 'true' 'REQ:SF103A_116' '' } %GIDa_9722da7d_caf8_4d5a_9cfd_9c770ef3705d  RndMeth=Zero
  Product1 : Product  RequirementInfo={'linktype_rmi_doors' '0000bb42 (/E-STEER Core/SubSystem Specifications/Application Functions/SF99/SF103A Motor Reference Model)' '#SF103A_116' 'true' 'REQ:SF103A_116' '' } %GIDa_f9f2a7c2_1abc_401b_b890_8df741651cac  RndMeth=Zero
  Subtract : Sum  RequirementInfo={'linktype_rmi_doors' '0000bb42 (/E-STEER Core/SubSystem Specifications/Application Functions/SF99/SF103A Motor Reference Model)' '#SF103A_116' 'true' 'REQ:SF103A_116' '' } %GIDa_e35af0c7_795b_4a18_89fa_762b54f57aac  Inputs=+-
  VdR_Amp : Outport  RequirementInfo={} %GIDa_bd7e0fa6_5c8e_406d_b215_4e5077d754ca
  VqR_Amp : Outport  RequirementInfo={} %GIDa_67912afd_0083_4a18_8b18_4dcaed93546b  Port=2
  wires:
  IqRef_Amp/1 -> Add/1, Product/1
  IdRef_Amp/1 -> Subtract/2, Product1/1
  IntermediateCalcs/1 -> Bus Selector1/1
  Bus Selector1/1 -> Product/2  "<ReacncQaxOverR>"
  Bus Selector1/2 -> Product1/2  "<ReacncDaxOverR>"
  Bus Selector1/3 -> Add/3  "<EgOverR_Ampr>"
  Product/1 -> Subtract/1
  Subtract/1 -> VdR_Amp/1
  Product1/1 -> Add/2
  Add/1 -> VqR_Amp/1

== system SF103A_MotRefMdl/MotRefMdl/MotRefMdlPer1/LocateRef/F_VoltTest_1 ==
  VdR_Amp : Inport  RequirementInfo={} %GIDa_7495eef0_9ee9_40d3_acad_7d93bc3530f2
  VqR_Amp : Inport  RequirementInfo={} %GIDa_86b00ad0_329e_4cea_83db_75ccd331d1ad  Port=2
  IntermediateCalcs : Inport  RequirementInfo={} %GIDa_22d83303_0b81_43eb_9a68_1e7b552a1708  Port=3
  Add : Sum  RequirementInfo={'linktype_rmi_doors' '0000bb42 (/E-STEER Core/SubSystem Specifications/Application Functions/SF99/SF103A Motor Reference Model)' '#SF103A_120' 'true' 'REQ:SF103A_120' '' } %GIDa_f2d3fcff_15d3_4ded_8c17_abda3dea2cbe
  Bus Selector1 : BusSelector  RequirementInfo={} %GIDa_0b013350_f372_43f2_9145_bb9f2924eb6c  OutputSignals=VovrRAllSqd_AmprSqd
  CopyRight2 : Subsystem  Description=|  mask(Copyright Information){none=on}
      | Copyright info block.                                               
      |                                                                     
      | Place copyright information at the top of every subsystem in design.
      mask prompts: none "No parameters"
      mask help: Place copyright information at the top of every subsystem in design.
      mask Display:
      | NxtrConf = 'Nexteer Confidential';
      | 
      | sys = bdroot; %handle for the current model ("system")
      | first = get_param(sys,'Created');
      | first = first(end-3:end);  %year is last four digits
      | 
      | last = get_param(sys,'LastModifiedDate');
      | if isempty(last)
      |     last = datestr(now,'yyyy');
      | else
      |     last = last(end-3:end);
      | end
      | 
      | if strcmp(first,last)
      |     fprintf('%s -- Copyright %s Nexteer',NxtrConf,first)
      | else
      |     fprintf('%s -- %s%s- %s Nexteer',NxtrConf,char(169),first,last)
      | end
  FALSE : Constant  RequirementInfo={'linktype_rmi_doors' '0000bb42 (/E-STEER Core/SubSystem Specifications/Application Functions/SF99/SF103A Motor Reference Model)' '#SF103A_120' 'true' 'REQ:SF103A_120' '' } %GIDa_d50ab4e9_ba1f_4435_97f0_a6de92bc949c  Value=false  OutDataTypeStr=boolean
  FALSE1 : Constant  RequirementInfo={'linktype_rmi_doors' '0000bb42 (/E-STEER Core/SubSystem Specifications/Application Functions/SF99/SF103A Motor Reference Model)' '#SF103A_120' 'true' 'REQ:SF103A_120' '' } %GIDa_a91be251_12b0_43a0_b56b_793e4c00f082  Value=true  OutDataTypeStr=boolean
  If : If  RequirementInfo={'linktype_rmi_doors' '0000bb42 (/E-STEER Core/SubSystem Specifications/Application Functions/SF99/SF103A Motor Reference Model)' '#SF103A_120' 'true' 'REQ:SF103A_120' '' } %GIDa_93c79568_cf0f_4c8f_8853_bac00d6e569f  NumInputs=2  IfExpression=u1 < u2
  Math Function : Math  RequirementInfo={'linktype_rmi_doors' '0000bb42 (/E-STEER Core/SubSystem Specifications/Application Functions/SF99/SF103A Motor Reference Model)' '#SF103A_120' 'true' 'REQ:SF103A_120' '' } %GIDa_2899248a_4962_4490_8cda_95ba7c81467b  Operator=square  SaturateOnIntegerOverflow=on
  Math Function1 : Math  RequirementInfo={'linktype_rmi_doors' '0000bb42 (/E-STEER Core/SubSystem Specifications/Application Functions/SF99/SF103A Motor Reference Model)' '#SF103A_120' 'true' 'REQ:SF103A_120' '' } %GIDa_9df1f75b_7b54_4461_bd84_7c2665cf077b  Operator=square  SaturateOnIntegerOverflow=on
  Merge : Merge  RequirementInfo={'linktype_rmi_doors' '0000bb42 (/E-STEER Core/SubSystem Specifications/Application Functions/SF99/SF103A Motor Reference Model)' '#SF103A_120' 'true' 'REQ:SF103A_120' '' } %GIDa_9873b338_0784_45a8_a91c_2275a60a3e15
  set_false : Subsystem  RequirementInfo={'linktype_rmi_doors' '0000bb42 (/E-STEER Core/SubSystem Specifications/Application Functions/SF99/SF103A Motor Reference Model)' '#SF103A_120' 'true' 'REQ:SF103A_120' '' } %GIDa_d9b5e3ca_df4c_4b33_a9b0_081b541f6c3f  TreatAsAtomicUnit=on
  set_true : Subsystem  RequirementInfo={'linktype_rmi_doors' '0000bb42 (/E-STEER Core/SubSystem Specifications/Application Functions/SF99/SF103A Motor Reference Model)' '#SF103A_120' 'true' 'REQ:SF103A_120' '' } %GIDa_59bdf322_00c1_4f9c_b95d_1c55b553a79d  TreatAsAtomicUnit=on
  VoltTest_Uls : Outport  RequirementInfo={} %GIDa_9619a6e3_dba1_4ee3_964e_21fc99742538
  wires:
  IntermediateCalcs/1 -> Bus Selector1/1
  Bus Selector1/1 -> If/2  "<VovrRAllSqd_AmprSqd>"
  VdR_Amp/1 -> Math Function/1  "VdR_Amp"
  VqR_Amp/1 -> Math Function1/1  "VqR_Amp"
  Math Function/1 -> Add/1
  Math Function1/1 -> Add/2
  Add/1 -> If/1  "Vdq_AmpSq"
  If/1 -> set_false/Action
  If/2 -> set_true/Action
  FALSE/1 -> set_false/1(In1)
  FALSE1/1 -> set_true/1(In1)
  set_false/1(Out1) -> Merge/1
  set_true/1(Out1) -> Merge/2
  Merge/1 -> VoltTest_Uls/1
